simulink model "thd_sim"  (R2015b)
settings: Solver=ode8  StartTime=0.0  StopTime=100e-3  FixedStep=1e-3  RelTol=1e-3
libraries: powerlib x1
settings Model: Creator=Aydin  LastModifiedBy=Aydin

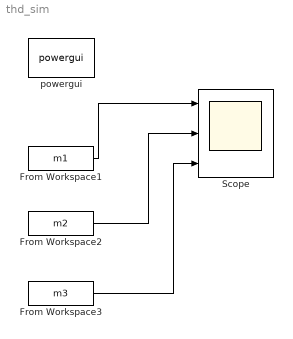
== system thd_sim ==
  From Workspace1 : FromWorkspace  VariableName=m1  SampleTime=0
  "From Workspace2 " : FromWorkspace  VariableName=m2  SampleTime=0
  From Workspace3 : FromWorkspace  VariableName=m3  SampleTime=0
  Scope : Scope  NumInputPorts=3
  powergui : powerlib/powergui  Priority=1  SimulationMode=Continuous  SolverType=Tustin/Backward Euler (TBE)  SampleTime=50e-6  frequency=60  SPID=off  DisableSnubberDevices=off  DisableRonSwitches=off  DisableVfSwitches=off  SwTol=0  DisplayEquations=off  Interpol=off  ExternalGateDelay=off  methode=off  Ts=10  FunctionMessages=off  echomessages=off  HookPort=off  EnableUseOfTLC=off  x0status=blocks  frequencyindice=60  Pbase=100e6  ErrMax=1e-4  Iterations=50  UnitsV=kV  UnitsW=MW  buscounter=0  RestoreLinks=warning  ResistiveCurrentMeasurement=off  Frange=[0:2:500]  Ylog=off  Xlog=on  ShowGrid=off  save=off  variable=ZData  structure=ScopeData  ZoomFFT=off  StartTime=0.0  cycles=2  DisplayStyle=2  fundamental=21.6  FreqAxis=off  MaxFrequency=500  frequencyindicesteady=1  RmsSteady=1  display=off
  wires:
  From Workspace1/1 -> Scope/1
  "From Workspace2 "/1 -> Scope/2
  From Workspace3/1 -> Scope/3
